simulink model "TST_InjCtl_qCoSync"  (R2016b)
settings: Solver=FixedStepDiscrete  StartTime=0.0  StopTime=3  FixedStep=sampleTime  RelTol=1e-3
values from neighbouring files (symbols this model uses):
  testCase = 1    [initTST_InjCtl_qCoSync_001.m]
libraries: simulink x3, UnitTest_Lib x1
settings Model: Creator=zhengjinyan  LastModifiedBy=zhengjinyan
settings DebuggingCC: SignalRangeChecking=error

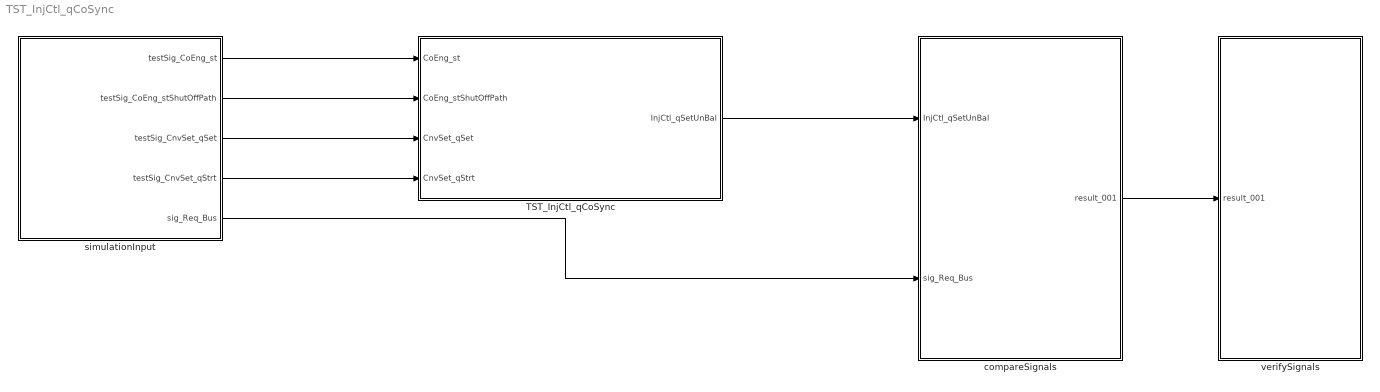
== system TST_InjCtl_qCoSync ==
  TST_InjCtl_qCoSync : Subsystem
  compareSignals : Subsystem
  simulationInput : Subsystem
  verifySignals : Subsystem
  wires:
  simulationInput/1(testSig_CoEng_st) -> TST_InjCtl_qCoSync/1(CoEng_st)
  simulationInput/2(testSig_CoEng_stShutOffPath) -> TST_InjCtl_qCoSync/2(CoEng_stShutOffPath)
  simulationInput/3(testSig_CnvSet_qSet) -> TST_InjCtl_qCoSync/3(CnvSet_qSet)
  simulationInput/4(testSig_CnvSet_qStrt) -> TST_InjCtl_qCoSync/4(CnvSet_qStrt)
  TST_InjCtl_qCoSync/1(InjCtl_qSetUnBal) -> compareSignals/1(InjCtl_qSetUnBal)
  simulationInput/5(sig_Req_Bus) -> compareSignals/2(sig_Req_Bus)
  compareSignals/1(result_001) -> verifySignals/1(result_001)

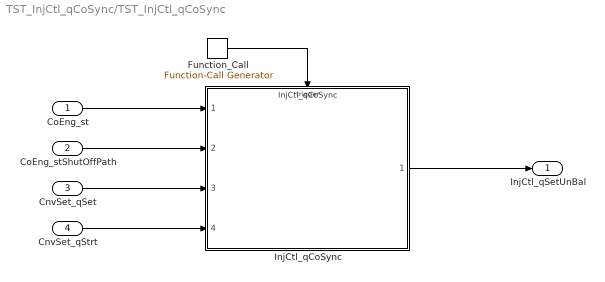
== system TST_InjCtl_qCoSync/TST_InjCtl_qCoSync ==
  CoEng_st : Inport
  CoEng_stShutOffPath : Inport  Port=2
  CnvSet_qSet : Inport  Port=3
  CnvSet_qStrt : Inport  Port=4
  Function_Call : simulink/Ports & Subsystems/Function-Call Generator  sample_time=sampleTime  numberOfIterations=1
  InjCtl_qCoSync : ModelReference  ModelNameDialog=InjCtl_qCoSync  SimulationMode=Normal  ModelReferenceVersion=1.7  TriggerPortName=function  TriggerPortTriggerType=function-call  TriggerPortStatesWhenEnabling=held
  InjCtl_qSetUnBal : Outport
  wires:
  Function_Call/1 -> InjCtl_qCoSync/Trigger
  CoEng_st/1 -> InjCtl_qCoSync/1
  CoEng_stShutOffPath/1 -> InjCtl_qCoSync/2
  CnvSet_qSet/1 -> InjCtl_qCoSync/3
  CnvSet_qStrt/1 -> InjCtl_qCoSync/4
  InjCtl_qCoSync/1 -> InjCtl_qSetUnBal/1

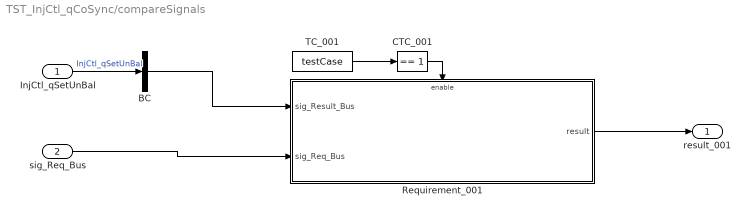
== system TST_InjCtl_qCoSync/compareSignals ==
  InjCtl_qSetUnBal : Inport
  sig_Req_Bus : Inport  Port=2
  BC : BusCreator  Inputs=1
  CTC_001 : simulink/Logic and Bit Operations/Compare To Constant  relop===  const=1  OutDataTypeStr=boolean
  Requirement_001 : Subsystem
  TC_001 : Constant  Value=testCase
  result_001 : Outport
  wires:
  InjCtl_qSetUnBal/1 -> BC/1  "InjCtl_qSetUnBal"
  TC_001/1 -> CTC_001/1
  CTC_001/1 -> Requirement_001/Enable
  sig_Req_Bus/1 -> Requirement_001/2(sig_Req_Bus)
  BC/1 -> Requirement_001/1(sig_Result_Bus)
  Requirement_001/1(result) -> result_001/1

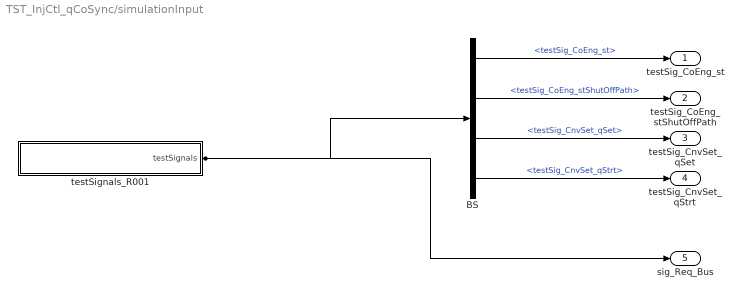
== system TST_InjCtl_qCoSync/simulationInput ==
  BS : BusSelector  OutputSignals=testSig_CoEng_st,testSig_CoEng_stShutOffPath,testSig_CnvSet_qSet,testSig_CnvSet_qStrt
  testSignals_R001 : Subsystem
  testSig_CoEng_st : Outport
  testSig_CoEng_stShutOffPath : Outport  Port=2
  testSig_CnvSet_qSet : Outport  Port=3
  testSig_CnvSet_qStrt : Outport  Port=4
  sig_Req_Bus : Outport  Port=5
  wires:
  BS/1 -> testSig_CoEng_st/1  "<testSig_CoEng_st>"
  BS/2 -> testSig_CoEng_stShutOffPath/1  "<testSig_CoEng_stShutOffPath>"
  BS/3 -> testSig_CnvSet_qSet/1  "<testSig_CnvSet_qSet>"
  BS/4 -> testSig_CnvSet_qStrt/1  "<testSig_CnvSet_qStrt>"
  testSignals_R001/1(testSignals) -> BS/1, sig_Req_Bus/1

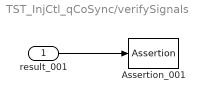
== system TST_InjCtl_qCoSync/verifySignals ==
  result_001 : Inport
  Assertion_001 : Assertion
  wires:
  result_001/1 -> Assertion_001/1

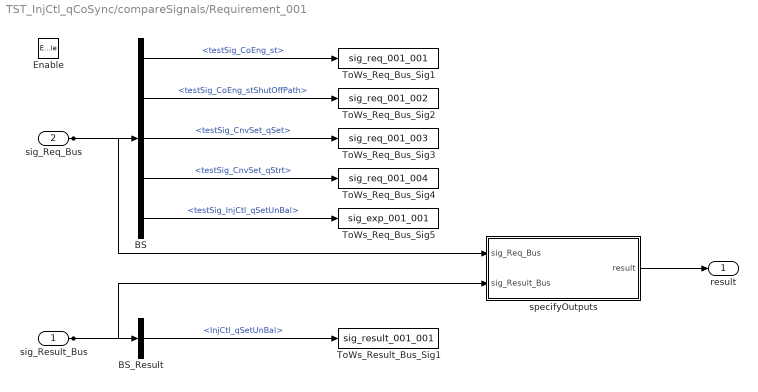
== system TST_InjCtl_qCoSync/compareSignals/Requirement_001 ==
  sig_Result_Bus : Inport
  sig_Req_Bus : Inport  Port=2
  Enable : EnablePort
  BS : BusSelector  OutputSignals=testSig_CoEng_st,testSig_CoEng_stShutOffPath,testSig_CnvSet_qSet,testSig_CnvSet_qStrt,testSig_InjCtl_qSetUnBal
  BS_Result : BusSelector  OutputSignals=InjCtl_qSetUnBal
  ToWs_Req_Bus_Sig1 : ToWorkspace  VariableName=sig_req_001_001  SaveFormat=Structure With Time
  ToWs_Req_Bus_Sig2 : ToWorkspace  VariableName=sig_req_001_002  SaveFormat=Structure With Time
  ToWs_Req_Bus_Sig3 : ToWorkspace  VariableName=sig_req_001_003  SaveFormat=Structure With Time
  ToWs_Req_Bus_Sig4 : ToWorkspace  VariableName=sig_req_001_004  SaveFormat=Structure With Time
  ToWs_Req_Bus_Sig5 : ToWorkspace  VariableName=sig_exp_001_001  SaveFormat=Structure With Time
  ToWs_Result_Bus_Sig1 : ToWorkspace  VariableName=sig_result_001_001  SaveFormat=Structure With Time
  specifyOutputs : Subsystem
  result : Outport
  wires:
  sig_Req_Bus/1 -> BS/1, specifyOutputs/1(sig_Req_Bus)
  BS/1 -> ToWs_Req_Bus_Sig1/1  "<testSig_CoEng_st>"
  BS/2 -> ToWs_Req_Bus_Sig2/1  "<testSig_CoEng_stShutOffPath>"
  BS/3 -> ToWs_Req_Bus_Sig3/1  "<testSig_CnvSet_qSet>"
  BS/4 -> ToWs_Req_Bus_Sig4/1  "<testSig_CnvSet_qStrt>"
  BS/5 -> ToWs_Req_Bus_Sig5/1  "<testSig_InjCtl_qSetUnBal>"
  sig_Result_Bus/1 -> BS_Result/1, specifyOutputs/2(sig_Result_Bus)
  BS_Result/1 -> ToWs_Result_Bus_Sig1/1  "<InjCtl_qSetUnBal>"
  specifyOutputs/1(result) -> result/1

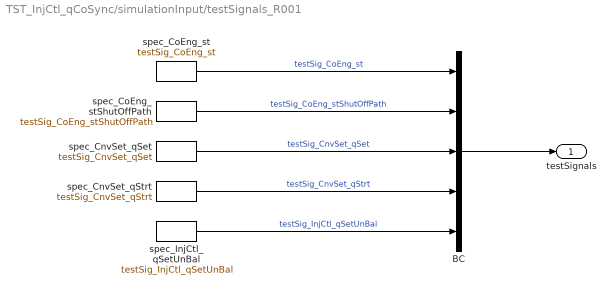
== system TST_InjCtl_qCoSync/simulationInput/testSignals_R001 ==
  BC : BusCreator  Inputs=5
  spec_CnvSet_qSet : FromWorkspace  VariableName=testSig_CnvSet_qSet  Interpolate=off  OutputAfterFinalValue=Holding final value
  spec_CnvSet_qStrt : FromWorkspace  VariableName=testSig_CnvSet_qStrt  Interpolate=off  OutputAfterFinalValue=Holding final value
  spec_CoEng_st : FromWorkspace  VariableName=testSig_CoEng_st  Interpolate=off  OutputAfterFinalValue=Holding final value
  spec_CoEng_stShutOffPath : FromWorkspace  VariableName=testSig_CoEng_stShutOffPath  Interpolate=off  OutputAfterFinalValue=Holding final value
  spec_InjCtl_qSetUnBal : FromWorkspace  VariableName=testSig_InjCtl_qSetUnBal  Interpolate=off  OutputAfterFinalValue=Holding final value
  testSignals : Outport
  wires:
  BC/1 -> testSignals/1
  spec_CoEng_st/1 -> BC/1  "testSig_CoEng_st"
  spec_CoEng_stShutOffPath/1 -> BC/2  "testSig_CoEng_stShutOffPath"
  spec_CnvSet_qSet/1 -> BC/3  "testSig_CnvSet_qSet"
  spec_CnvSet_qStrt/1 -> BC/4  "testSig_CnvSet_qStrt"
  spec_InjCtl_qSetUnBal/1 -> BC/5  "testSig_InjCtl_qSetUnBal"

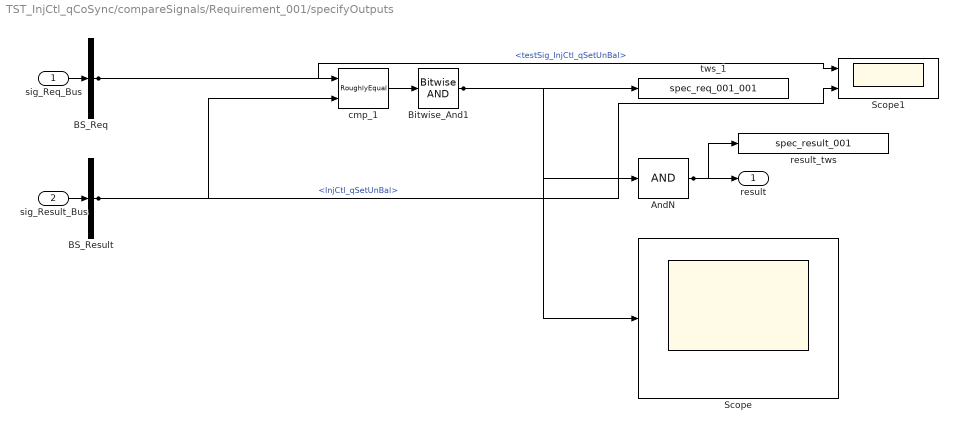
== system TST_InjCtl_qCoSync/compareSignals/Requirement_001/specifyOutputs ==
  sig_Req_Bus : Inport
  sig_Result_Bus : Inport  Port=2
  AndN : Logic  Inputs=1
  BS_Req : BusSelector  OutputSignals=testSig_InjCtl_qSetUnBal
  BS_Result : BusSelector  OutputSignals=InjCtl_qSetUnBal
  Bitwise_And1 : simulink/Logic and Bit Operations/Bitwise Operator  logicop=AND  UseBitMask=off  BitMask=bin2dec('11011001')  BitMaskRealWorld=Stored Integer
  Scope : Scope
  Scope1 : Scope  NumInputPorts=2
  cmp_1 : UnitTest_Lib/RoughlyEqual  slope=0.1
  result_tws : ToWorkspace  VariableName=spec_result_001
  tws_1 : ToWorkspace  VariableName=spec_req_001_001
  result : Outport
  wires:
  sig_Req_Bus/1 -> BS_Req/1
  sig_Result_Bus/1 -> BS_Result/1
  AndN/1 -> result/1, result_tws/1
  BS_Req/1 -> cmp_1/1, Scope1/1  "<testSig_InjCtl_qSetUnBal>"
  BS_Result/1 -> cmp_1/2, Scope1/2  "<InjCtl_qSetUnBal>"
  cmp_1/1 -> Bitwise_And1/1
  Bitwise_And1/1 -> tws_1/1, AndN/1, Scope/1
